simulink model "M3"  (R2012b)
settings: Solver=ode45  StartTime=0.0  StopTime=8  RelTol=1e-3
libraries: simulink x2
settings Model: Creator=user  LastModifiedBy=user
settings DebuggingCC: SolverPrmCheckMsg=none

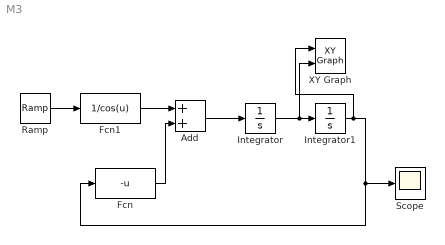
== system M3 ==
  Add : Sum
  Fcn : Fcn  Expr=-u
  Fcn1 : Fcn  Expr=1/cos(u)
  Integrator : Integrator
  Integrator1 : Integrator
  Ramp : simulink/Sources/Ramp  slope=1  start=0  X0=0
  Scope : Scope
  XY Graph : simulink/Sinks/XY Graph  xmin=-10  xmax=10  ymin=-10  ymax=10  st=-1
  wires:
  Ramp/1 -> Fcn1/1
  Fcn/1 -> Add/2
  Fcn1/1 -> Add/1
  Add/1 -> Integrator/1
  Integrator/1 -> XY Graph/2, Integrator1/1
  Integrator1/1 -> XY Graph/1, Scope/1, Fcn/1
